simulink model "lab5_model_2012b"  (R2012b)
settings: Solver=ode45  StartTime=0.0  StopTime=100  RelTol=1e-3
values from neighbouring files (symbols this model uses):
  D = 52    [lab5.m]
  K = 100    [lab5.m]
  M1 = 1000    [lab5.m]
  M2 = 1500    [lab5.m]
settings Model: Creator=Jessica  LastModifiedBy=Jessica
settings OptimizationCC: ExpressionDepthLimit=128
settings DebuggingCC: UnderspecifiedInitializationDetection=Simplified  MergeDetectMultiDrivingBlocksExec=error  SolverPrmCheckMsg=none  FrameProcessingCompatibilityMsg=error  StateNameClashWarn=none
settings CodeAppCC: CustomSymbolStrType=$N$R$M_T
settings GRTTargetCC: CodeReplacementLibrary=C89/C90 (ANSI)

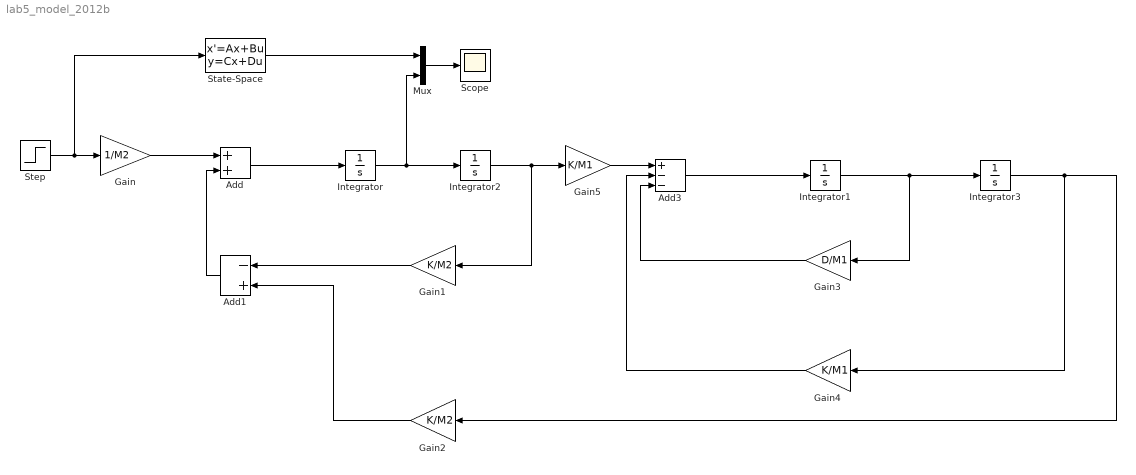
== system lab5_model_2012b ==
  Add : Sum
  Add1 : Sum  Inputs=-+
  Add3 : Sum  Inputs=+--
  Gain : Gain  Gain=1/M2
  Gain1 : Gain  Gain=K/M2
  Gain2 : Gain  Gain=K/M2
  Gain3 : Gain  Gain=D/M1
  Gain4 : Gain  Gain=K/M1
  Gain5 : Gain  Gain=K/M1
  Integrator{,1..3} (4 alike) : Integrator
  Mux : Mux  Inputs=2
  Scope : Scope
      settings: SaveName=y
  State-Space : StateSpace  A=[0 1 0 0;(-K/M1) (-D/M1) (K/M1) 0;0 0 0 1;(K/M2) 0 (-K/M2) 0]  B=[0;0;0;(1/M2)]  C=[0 0 0 1]  D=0  X0=0
  Step : Step  Before=1  After=0  SampleTime=0
  wires:
  Gain/1 -> Add/1
  Add1/1 -> Add/2
  Add/1 -> Integrator/1
  Gain1/1 -> Add1/1
  Gain2/1 -> Add1/2
  Add3/1 -> Integrator1/1
  Integrator1/1 -> Gain3/1, Integrator3/1
  Integrator3/1 -> Gain2/1, Gain4/1
  Gain5/1 -> Add3/1
  Integrator2/1 -> Gain1/1, Gain5/1
  Integrator/1 -> Mux/2, Integrator2/1
  Step/1 -> State-Space/1, Gain/1
  Mux/1 -> Scope/1
  State-Space/1 -> Mux/1
  Gain3/1 -> Add3/3
  Gain4/1 -> Add3/2
